simulink model "do178b_dhc2_rev1"  (R2018a)
settings: Solver=ode23  StartTime=0.0  StopTime=25  MaxStep=1/40  RelTol=1e-2  AbsTol=1e-3  EnableMultiTasking=on
PreLoadFcn:
  | load asbdhc2_init;
  | Autopilot_bus;
model workspace (MAT data in the model file):
  ALT_Mode = [0 0 0 0 0 0 0 0 0 0 0 0 ... (1001 elements, 1001x1)]
  ALT_Ref = [991.703720962 991.703720962 991.703720962 991.703720962 991.703720962 991.703720962 991.703720962 991.703720962 991.703720962 991.703720962 991.703720962 991.703720962 ... (1001 elements, 1001x1)]
  AP_Eng = [1 1 1 1 1 1 1 1 1 1 1 1 ... (1001 elements, 1001x1)]
  AilCmdv = [0; 0; 0]
  MCOS : class17 (value not decoded)
  FR = [0; 0]
  Ft = [0 0.333333333333 0.333333333333 0.333333333333 0.333333333333 0.333333333333 0.333333333333 0.333333333333 0.333333333333 0.333333333333 0.333333333333 0.333333333333 ... (1001 elements, 1001x1)]
  HDG_Mode = [0 0 0 0 0 0 0 0 0 0 0 0 ... (1001 elements, 1001x1)]
  HDG_Ref = [29.7066688805 29.7066688805 29.7066688805 29.7066688805 29.7066688805 29.7066688805 29.7066688805 29.7066688805 29.7066688805 29.7066688805 29.7066688805 29.7066688805 ... (1001 elements, 1001x1)]
  InputSize = 2
  N = 37
  PhiRefv = [0; 0; 0]
  MCOS : class17 (value not decoded)
  Phiv = [0; 0; 0]
  Pwheel = [2.59796598511 2.59796598511 2.59796598511 2.59796598511 2.59796598511 2.59796598511 2.59796598511 2.59796598511 2.59796598511 2.59796598511 2.59796598511 2.59796598511 ... (1001 elements, 1001x1)]
  Roll_Mode = [1 1 1 1 1 1 1 1 1 1 1 1 ... (1001 elements, 1001x1)]
  TimeSteps = 1001
  Tkv = [0; 0; 0]
  TurnK = [-15.9132354515 -15.9132354515 -15.9132354515 -15.9132354515 -15.9132354515 -15.9132354515 -15.9132354515 -15.9132354515 -15.9132354515 -15.9132354515 -15.9132354515 -15.9132354515 ... (1001 elements, 1001x1)]
  X = [0 0 1 0 1 1 1 0 0 -58.6358480164 -121.61436905 105.942434646 ... (21 elements, 1x21)]
  a = -2.96750408985
  a1 = [11.3528701884 11.3528701884 11.3528701884 11.3528701884 11.3528701884 11.3528701884 11.3528701884 11.3528701884 11.3528701884 11.3528701884 11.3528701884 11.3528701884 ... (1001 elements, 1x1001)]
  apin : struct (value not decoded)
  apsin : struct (value not decoded)
  curPath = '/Users/khouloud.gaaloul/Documents/Projects/QRA-LocalSearch/Local Search Algorithms/Problems'
  d = 22
  MCOS : class17 (value not decoded)
  i = 9
  inertial : struct (value not decoded)
  j = 7
  list : struct (value not decoded)
  modelpath = '/Users/khouloud.gaaloul/Documents/Projects/QRA-LocalSearch/Simulink Models/autopilot/aprevised/'
  models : cell (value not decoded)
  n = 1
  nbrInputs = 7
  req = 'R1.4.2'
  rollOut = []
  MCOS : class17 (value not decoded)
  t = [0 0.025 0.05 0.075 0.1 0.125 0.15 0.175 0.2 0.225 0.25 0.275 ... (1001 elements, 1x1001)]
undefined symbols (not defined in the file): beaver_b, beaver_c, beaver_init_p, beaver_init_pitch, beaver_init_q, beaver_init_r, beaver_init_roll, beaver_mass, Cl0, Cl_alpha2_dpt, Cl_beta, Cl_da, Cl_da_alpha, Cl_dr, Cl_p, Cl_r, Cm0, Cm_alpha, Cm_alpha2, Cm_beta2, Cm_de, Cm_df, Cm_dpt, Cm_q, Cm_r, Cn0, Cn_beta, Cn_beta3, Cn_da, Cn_dpt3, Cn_dr, Cn_p, Cn_q, Cn_r, Cx0, Cx_alpha, Cx_alpha2, Cx_alpha3, Cx_df, Cx_df_alpha, Cx_dpt, Cx_dpt2_alpha, Cx_dr, Cx_q, Cy0, Cy_beta, Cy_da, Cy_dr, Cy_dr_alpha, Cy_p, Cy_r, Cz0, Cz_alpha, Cz_alpha3, Cz_de, Cz_de_beta, Cz_df, Cz_df_alpha, Cz_dpt, Cz_q ... (+9)
libraries: aerolibconvert2 x6, simulink x6, aerolibobsolete x5, aerolibasang x3, aerolibwind2 x3, aerolibadyn x1, aerolibatmos2 x1
(part 3 of 3)

== system do178b_dhc2_rev1/DeHavilland Beaver Airframe/Aircraft Dynamics/Total Forces and Moments/Aerodynamics/Body Rate Damping/p ==
  Constant1 : Constant  Value=0
  Constant2 : Constant  Value=Cy_p
  Constant3 : Constant  Value=Cl_p
  Constant4 : Constant  Value=Cn_p
  Mux1 : Mux  Inputs=6
  delCoeff : Outport
  wires:
  Constant2/1 -> Mux1/2
  Mux1/1 -> delCoeff/1
  Constant1/1 -> Mux1/5, Mux1/3, Mux1/1
  Constant4/1 -> Mux1/6
  Constant3/1 -> Mux1/4

== system do178b_dhc2_rev1/DeHavilland Beaver Airframe/Aircraft Dynamics/Total Forces and Moments/Aerodynamics/Body Rate Damping/q ==
  Constant1 : Constant  Value=0
  Constant2 : Constant  Value=Cz_q
  Constant3 : Constant  Value=Cx_q
  Constant4 : Constant  Value=Cm_q
  Constant5 : Constant  Value=Cn_q
  Mux1 : Mux  Inputs=6
  delCoeff : Outport
  wires:
  Constant2/1 -> Mux1/3
  Constant5/1 -> Mux1/6
  Constant1/1 -> Mux1/4, Mux1/2
  Constant4/1 -> Mux1/5
  Constant3/1 -> Mux1/1
  Mux1/1 -> delCoeff/1

== system do178b_dhc2_rev1/DeHavilland Beaver Airframe/Aircraft Dynamics/Total Forces and Moments/Aerodynamics/Body Rate Damping/r ==
  Constant : Constant  Value=0
  Constant1 : Constant  Value=Cy_r
  Constant2 : Constant  Value=Cl_r
  Constant3 : Constant  Value=Cm_r
  Constant4 : Constant  Value=Cn_r
  Mux1 : Mux  Inputs=6
  delCoeff : Outport
  wires:
  Constant3/1 -> Mux1/5
  Constant1/1 -> Mux1/2
  Constant4/1 -> Mux1/6
  Constant2/1 -> Mux1/4
  Constant/1 -> Mux1/3, Mux1/1
  Mux1/1 -> delCoeff/1
